simulink model "PV_fed_VCIMD_updated"  (R2019a)
settings: Solver=FixedStepAuto  StartTime=0.0  StopTime=20  RelTol=1e-3
undefined symbols (not defined in the file): L, Lm, Lr, Rr, sigbuilder_block
libraries: powerlib_meascontrol x17, powerlib x16, re_lib x1
settings Model: SimulationMode=accelerator  Creator=jetha  LastModifiedBy=HP
settings DataIOCC: ReturnWorkspaceOutputs=off
settings DebuggingCC: ArithmeticOperatorsInVariantConditions=warning

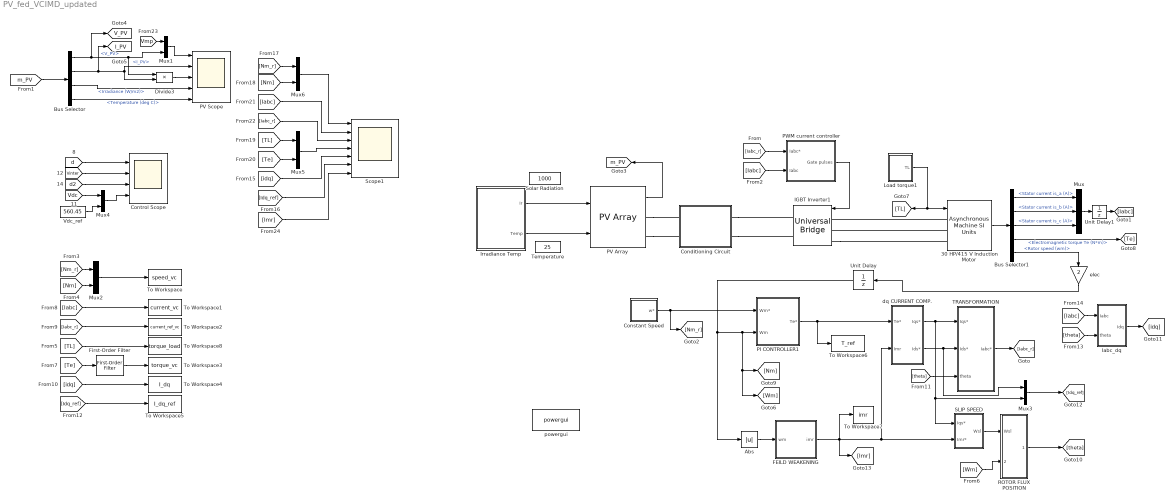
== system PV_fed_VCIMD_updated ==
  30 HP/415 V Induction Motor : powerlib/Machines/Asynchronous Machine SI Units  RotorType=Squirrel-cage  PresetModel=No  MechanicalLoad=Torque Tm  ShowDetailedParameters=on  ReferenceFrame=Rotor  Units=SI  MeasurementBus=off  NominalParameters=[30*746 415 50]  Stator=[0.251 0.001397]  Rotor=[Rr 0.001397]  Cage1=[ 0.022 0.226/377]  Cage2=[ 0.022 0.226/377]  Lm=0.0416  Mechanical=[0.305 0 2 ]  PolePairs=2  InitialConditions=[1 0 0 0 0 0 0 0]  SimulateSaturation=off  Saturation=[14.03593122, 27.81365428, 53.79336849, 72.68890987, 97.98006896, 148.6815601, 215.7428561, 302.9841135, 420.4778367 ; 230, 322, 414, 460, 506, 552, 598, 644, 690]  LoadFlowParameters=1492000  TsPowergui=0  TsBlock=-1  IterativeModel=Trapezoidal non iterative  IterativeDiscreteModel=Trapezoidal non iterative  Pmec=0
      settings: SourceProductName=Simscape Electrical
  Abs : Abs  SaturateOnIntegerOverflow=on
  Bus Selector : BusSelector  OutputSignals=V_PV,I_PV,Irradiance (W/m2),Temperature (deg C)
  Bus Selector1 : BusSelector  OutputSignals=Stator measurements.Stator current is_a (A),Stator measurements.Stator current is_b (A),Stator measurements.Stator current is_c (A),Mechanical.Electromagnetic torque Te (N*m),Mechanical.Rotor speed (wm)
  Conditioning Circuit : Subsystem
  Constant Speed : Subsystem
  Control Scope : Scope  NumInputPorts=4
  Divide3 : Product  Inputs=**
  FEILD WEAKENING : MATLAB Function  TreatAsAtomicUnit=on
  First-Order Filter : powerlib_meascontrol/Filters/First-Order Filter  FilterType=Lowpass  Tc=10e-3  Ts=0  Initialize=on  Vac_Init=[0, 0, 60]  Vdc_Init=0  PlotResponse=off  FreqRange="[0,  200,  1]"
      settings: SourceProductName=Simscape Electrical
  IGBT Inverter1 : powerlib/Power Electronics/Universal Bridge  Arms=3  SnubberResistance=1e5  SnubberCapacitance=inf  Device=MOSFET / Diodes  Ron=1e-3  Lon=0  ForwardVoltages="[  0  0  ]"  ForwardVoltage=0  GTOparameters=[ 10e-6 , 20e-6 ]  IGBTparameters=[ 1e-6 , 2e-6 ]  Measurements=None  Measurements_2=None  converterType=Rectifier
      settings: SourceProductName=Simscape Electrical
  Iabc_dq : Subsystem
  Irradiance Temp : Subsystem  Tag=STV Subsys  LoadFcn=sigbuilder_block('load');  StartFcn=sigbuilder_block('start');  StopFcn=sigbuilder_block('stop');  ClipboardFcn=sigbuilder_block('clipboard');  mask(Sigbuilder block){tuvar=[0:10]}
      mask help: Sigbuilder GUI
      mask init:
      | if ~strcmp(get_param(bdroot(gcbh),'SimulationStatus'),'stopped') tuvar = sigbuilder_block('maskInit'); end
      settings: CopyFcn=sigbuilder_block('copy');  DeleteFcn=sigbuilder_block('delete');  ModelCloseFcn=sigbuilder_block('modelClose');  PreSaveFcn=sigbuilder_block('preSave');  PauseFcn=sigbuilder_block('pause')  ContinueFcn=sigbuilder_block('continue')  NameChangeFcn=sigbuilder_block('namechange');  OpenFcn=sigbuilder_block('open',[87 109.8 1012.8 447.6 ]);  CloseFcn=sigbuilder_block('close');
      mask Display: plot(0, 0, 100, 100,[2, 2, 32, 32, 2], [68, 8, 8, 68, 68],[32, 2], [38, 38], [32, 19, 2],[53, 60, 44], [32, 17, 17, 2],[16, 16, 31, 31]);txt = getActiveGroup(gcbh);text(2, 100, txt,'verticalAlignment', 'top');
  Load torque1 : Subsystem
  Mux : Mux  Inputs=3
  Mux{1..6} (6 alike) : Mux  Inputs=2
  PI CONTROLLER1 : Subsystem  mask{Kp=120, Ki=2, Ts=100e-6, Lim=500}
      mask prompts: Ts "Sampling Time Ts (sec)"; Lim "Ref Torque limit(N-m)"
  PV Array : re_lib/Solar/PV Array  Npar=5  Nser=20  PlotType=array @ 25 deg.C & specified irradiances  S_vec=[ 1000 500 250 100 ]  Temp_C_vec="[ 25  50]"  ModuleName=Waaree Energies WSM-315  PlotWhenSelected=off  Pm=315  Ncell=72  Voc=43  Isc=9.77  Vm=35  Im=9  beta_Voc_pc=-0.338  alpha_Isc_pc=0.040901  beta_Voc=-0.14534  alpha_Isc=0.003996  IL=9.7966  I0=1.447e-10  nI=0.93356  Rsh=115.0566  Rs=0.31273  BAL=on  Tc=1e-6  Tfilter=5e-6
      settings: SourceProductName=Simscape Electrical
  PV Scope : Scope  NumInputPorts=5
  PWM current controller : Subsystem
  ROTOR FLUX POSITION : Subsystem
  SLIP SPEED : Subsystem
  Scope1 : Scope  NumInputPorts=7
  Solar Radiation : Constant  Value=1000
  TRANSFORMATION : Subsystem
  Temperature : Constant  Value=25
  To Workspace : ToWorkspace  VariableName=speed_vc  SaveFormat=Structure With Time  SampleTime=100e-6
  To Workspace1 : ToWorkspace  VariableName=current_vc  SaveFormat=Structure With Time  SampleTime=100e-6
  To Workspace2 : ToWorkspace  VariableName=current_ref_vc  SaveFormat=Structure With Time  SampleTime=100e-6
  To Workspace3 : ToWorkspace  VariableName=torque_vc  SaveFormat=Structure With Time  SampleTime=100e-6
  To Workspace4 : ToWorkspace  VariableName=I_dq  SaveFormat=Structure With Time  SampleTime=100e-6
  To Workspace5 : ToWorkspace  VariableName=I_dq_ref  SaveFormat=Structure With Time  SampleTime=100e-6
  To Workspace6 : ToWorkspace  VariableName=T_ref  SaveFormat=Structure With Time  SampleTime=100e-6
  To Workspace7 : ToWorkspace  VariableName=imr  SaveFormat=Structure With Time  SampleTime=100e-6
  To Workspace8 : ToWorkspace  VariableName=torque_load  SaveFormat=Structure With Time  SampleTime=100e-6
  Unit Delay : UnitDelay  SampleTime=100e-6  HasFrameUpgradeWarning=on
  Unit Delay1 : UnitDelay  SampleTime=10e-6  HasFrameUpgradeWarning=on
  Vdc_ref : Constant  Value=560.45
  dq CURRENT COMP. : Subsystem
  elec : Gain  Gain=2
  powergui : powerlib/powergui  Priority=1  SimulationMode=Discrete  SampleTime=1e-5  frequency=60  Iterations=50  frequencyindice=0  Pbase=100e6  ErrMax=1e-4  UnitsV=kV  UnitsW=MW  buscounter=0  FunctionMessages=off  echomessages=off  EnableUseOfTLC=off  CurrentSourceSwitches=off  DisableSnubberDevices=off  DisableRonSwitches=off  DisableVfSwitches=off  DisplayEquations=off  AutomaticDiscreteSolvers=off  SolverType=Tustin/Backward Euler (TBE)  Interpol=off  ExternalGateDelay=off  methode=off  Ts=100  x0status=blocks  SPID=off  SwTol=0  HookPort=off  NonlinearTolerance=0  nMaxIteration=15  ContinueOnMaxIteration=off  RestoreLinks=warning  ResistiveCurrentMeasurement=off  Frange=[0:2:500]  Ylog=off  Xlog=on  ShowGrid=off  save=off  variable=ZData  structure=0  ZoomFFT=off  StartTime=0.0  cycles=1  DisplayStyle=1  fundamental=60  FreqAxis=off  MaxFrequency=1000  frequencyindicesteady=1  RmsSteady=1  display=off
      settings: SourceProductName=Simscape Electrical
  tag scope: I_PV=global, V_PV=global, m_PV=global
  wires:
  PV Array/1 -> [m_PV]
  Load torque1/1(TL) -> 30 HP/415 V Induction Motor/1, [TL]
  [theta] -> Iabc_dq/2(theta)
  [Iabc] -> Iabc_dq/1(Iabc)
  SLIP SPEED/1(Wsl) -> ROTOR FLUX POSITION/1("Wsl\t")
  elec/1 -> Unit Delay/1
  [theta] -> TRANSFORMATION/3(theta)
  [Iabc_r] -> PWM current controller/1(Iabc*)
  [Wm] -> ROTOR FLUX POSITION/2(Wm)
  Bus Selector1/4 -> [Te]  "<Electromagnetic torque Te (N*m)>"
  ROTOR FLUX POSITION/1(theta) -> [theta]
  dq CURRENT COMP./1(Iqs*) -> TRANSFORMATION/1(Iqs*), SLIP SPEED/1(Iqs*), Mux3/2
  Mux3/1 -> [Idq_ref]
  Abs/1 -> FEILD WEAKENING/1(wm)
  Unit Delay1/1 -> [Iabc]
  Iabc_dq/1(Idq) -> [idq]
  PWM current controller/1(Gate pulses) -> IGBT Inverter1/1
  Bus Selector1/5 -> elec/1  "<Rotor speed (wm)>"
  30 HP/415 V Induction Motor/1 -> Bus Selector1/1
  Mux/1 -> Unit Delay1/1
  dq CURRENT COMP./2(Ids*) -> Mux3/1, TRANSFORMATION/2(Ids*)
  Bus Selector1/1 -> Mux/1  "<Stator current is_a (A)>"
  FEILD WEAKENING/1(imr) -> [Imr], dq CURRENT COMP./2(Imr), SLIP SPEED/2(Imr*), To Workspace7/1
  Unit Delay/1 -> Abs/1, PI CONTROLLER1/2(Wm), [Nm], [Wm]
  Bus Selector1/2 -> Mux/2  "<Stator current is_b (A)>"
  TRANSFORMATION/1(Iabc*) -> [Iabc_r]
  PI CONTROLLER1/1(Te*) -> To Workspace6/1, dq CURRENT COMP./1(Te*)
  Bus Selector1/3 -> Mux/3  "<Stator current is_c (A)>"
  [Iabc] -> PWM current controller/2(Iabc)
  Constant Speed/1(w*) -> PI CONTROLLER1/1(Wm*), [Nm_r]
  Irradiance Temp/1(Ir) -> PV Array/1
  Irradiance Temp/2(Temp) -> PV Array/2
  [d] -> Control Scope/1
  [Iabc] -> Scope1/2
  [Te] -> First-Order Filter/1
  Mux2/1 -> To Workspace/1
  [Iabc] -> To Workspace1/1
  [Nm] -> Mux2/2
  Vdc_ref/1 -> Mux4/2
  Mux4/1 -> Control Scope/4
  Mux5/1 -> Scope1/4
  [Idq_ref] -> To Workspace5/1
  Bus Selector/3 -> PV Scope/4  "<Irradiance (W/m2)>"
  [Vdc] -> Mux4/1
  Mux1/1 -> PV Scope/1
  [idq] -> Scope1/5
  Bus Selector/2 -> [I_PV], PV Scope/2, Divide3/2  "<I_PV>"
  [d2] -> Control Scope/3
  Divide3/1 -> PV Scope/3
  [TL] -> To Workspace8/1
  [Te] -> Mux5/2
  Bus Selector/4 -> PV Scope/5  "<Temperature (deg C)>"
  [TL] -> Mux5/1
  [Nm] -> Mux6/2
  [m_PV] -> Bus Selector/1
  Mux6/1 -> Scope1/1
  [Iabc_r] -> Scope1/3
  Bus Selector/1 -> [V_PV], Mux1/2, Divide3/1  "<V_PV>"
  [idq] -> To Workspace4/1
  [Iabc_r] -> To Workspace2/1
  [Idq_ref] -> Scope1/6
  [Nm_r] -> Mux2/1
  First-Order Filter/1 -> To Workspace3/1
  [Nm_r] -> Mux6/1
  [Vinter] -> Control Scope/2
  [Vmp] -> Mux1/1
  [Imr] -> Scope1/7
  connections:
  PV Array/RConn1 -- Conditioning Circuit/LConn1
  PV Array/RConn2 -- Conditioning Circuit/LConn2
  30 HP/415 V Induction Motor/LConn1 -- IGBT Inverter1/LConn1
  IGBT Inverter1/LConn3 -- 30 HP/415 V Induction Motor/LConn3
  30 HP/415 V Induction Motor/LConn2 -- IGBT Inverter1/LConn2
  Conditioning Circuit/RConn1 -- IGBT Inverter1/RConn1
  Conditioning Circuit/RConn2 -- IGBT Inverter1/RConn2

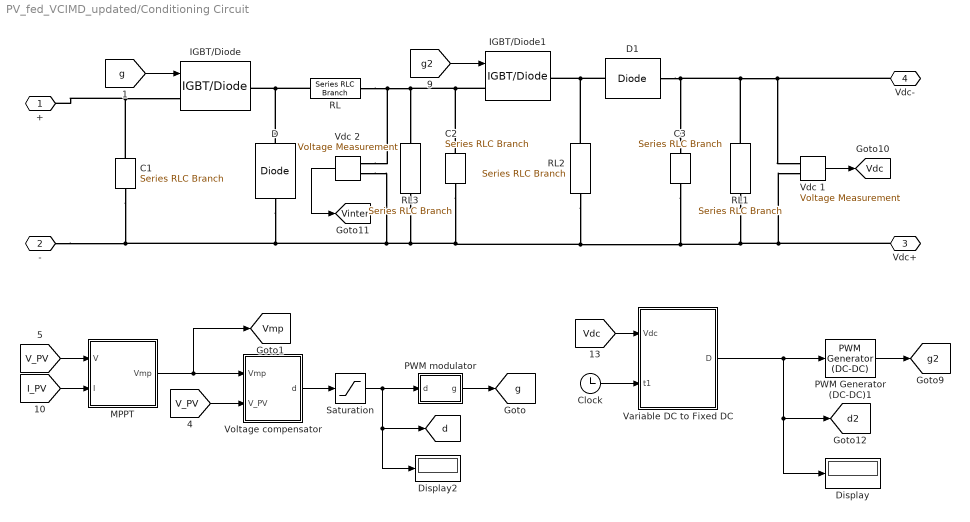
== system PV_fed_VCIMD_updated/Conditioning Circuit ==
  C1 : powerlib/Elements/Series RLC Branch  LConnTagsString=__new0  RConnTagsString=__new0  BranchType=C  Resistance=1  Inductance=L  SetiL0=off  InitialCurrent=0  Capacitance=1e-3  Setx0=off  InitialVoltage=Vmp  Measurements=None
      settings: SourceProductName=Simscape Electrical
  C2 : powerlib/Elements/Series RLC Branch  LConnTagsString=__new0  RConnTagsString=__new0  BranchType=C  Resistance=1  Inductance=L  SetiL0=off  InitialCurrent=0  Capacitance=5e-3  Setx0=off  InitialVoltage=Vmp  Measurements=None
      settings: SourceProductName=Simscape Electrical
  C3 : powerlib/Elements/Series RLC Branch  LConnTagsString=__new0  RConnTagsString=__new0  BranchType=C  Resistance=1  Inductance=L  SetiL0=off  InitialCurrent=0  Capacitance=5e-2  Setx0=off  InitialVoltage=Vmp  Measurements=None
      settings: SourceProductName=Simscape Electrical
  Clock : Clock
  D : powerlib/Power Electronics/Diode  Ron=1e-4  Lon=0  Vf=0  IC=0  UseSnubber=off  Rs=inf  Cs=inf  Measurements=off
      settings: SourceProductName=Simscape Electrical
  D1 : powerlib/Power Electronics/Diode  Ron=1e-4  Lon=0  Vf=0  IC=0  UseSnubber=off  Rs=inf  Cs=inf  Measurements=off
      settings: SourceProductName=Simscape Electrical
  Display : Display
  Display2 : Display
  IGBT/Diode : powerlib/Power Electronics/IGBT//Diode  Ron=1e-3  Rs=1e5  Cs=inf  Measurements=off
      settings: SourceProductName=Simscape Electrical
  IGBT/Diode1 : powerlib/Power Electronics/IGBT//Diode  Ron=1e-3  Rs=1e5  Cs=inf  Measurements=off
      settings: SourceProductName=Simscape Electrical
  MPPT : MATLAB Function  TreatAsAtomicUnit=on
  PWM modulator : Subsystem
  PWM Generator (DC-DC)1 : powerlib_meascontrol/Pulse & Signal Generators/PWM Generator (DC-DC)  Fsw=10000  Ts=0
      settings: SourceProductName=Simscape Electrical
  RL : powerlib/Elements/Series RLC Branch  LConnTagsString=__new0  RConnTagsString=__new0  BranchType=RL  Resistance=5e-3  Inductance=0.01  SetiL0=off  InitialCurrent=0  Capacitance=1e-6  Setx0=off  InitialVoltage=0  Measurements=None
      settings: SourceProductName=Simscape Electrical
  RL1 : powerlib/Elements/Series RLC Branch  LConnTagsString=__new0  RConnTagsString=__new0  BranchType=R  Resistance=150  Inductance=10e-3  SetiL0=off  InitialCurrent=0  Capacitance=1e-6  Setx0=off  InitialVoltage=0  Measurements=None
      settings: SourceProductName=Simscape Electrical
  RL2 : powerlib/Elements/Series RLC Branch  LConnTagsString=__new0  RConnTagsString=__new0  BranchType=RL  Resistance=5e-3  Inductance=1e-2  SetiL0=off  InitialCurrent=0  Capacitance=1e-6  Setx0=off  InitialVoltage=0  Measurements=None
      settings: SourceProductName=Simscape Electrical
  RL3 : powerlib/Elements/Series RLC Branch  LConnTagsString=__new0  RConnTagsString=__new0  BranchType=R  Resistance=5  Inductance=10e-3  SetiL0=off  InitialCurrent=0  Capacitance=1e-6  Setx0=off  InitialVoltage=0  Measurements=None
      settings: SourceProductName=Simscape Electrical
  Saturation : Saturate  UpperLimit=0.9  LowerLimit=0.1  LinearizeAsGain=off
  Variable DC to Fixed DC : MATLAB Function  TreatAsAtomicUnit=on
  Vdc 1 : powerlib/Measurements/Voltage Measurement  Tag=PoWeRsYsTeMmEaSuReMeNt  PhasorSimulation=off  OutputType=Magnitude  PSBequivalent=0
      settings: SourceProductName=Simscape Electrical
  Vdc 2 : powerlib/Measurements/Voltage Measurement  Tag=PoWeRsYsTeMmEaSuReMeNt  PhasorSimulation=off  OutputType=Magnitude  PSBequivalent=0
      settings: SourceProductName=Simscape Electrical
  Voltage compensator : Subsystem
  + : PMIOPort  Side=Left
  - : PMIOPort  Port=2  Side=Left
  Vdc+ : PMIOPort  Port=3  Side=Right
  Vdc- : PMIOPort  Port=4  Side=Right
  tag scope: Vdc=global, Vinter=global, Vmp=global, d2=global, d=global, g2=global, g=global
  wires:
  PWM Generator (DC-DC)1/1 -> [g2]
  [Vdc] -> Variable DC to Fixed DC/1(Vdc)
  Variable DC to Fixed DC/1(D) -> Display/1, [d2], PWM Generator (DC-DC)1/1
  Clock/1 -> Variable DC to Fixed DC/2(t1)
  [V_PV] -> Voltage compensator/2(V_PV)
  [I_PV] -> MPPT/2(I)
  [V_PV] -> MPPT/1(V)
  PWM modulator/1(g) -> [g]
  MPPT/1(Vmp) -> [Vmp], Voltage compensator/1(Vmp)
  Voltage compensator/1(d) -> Saturation/1
  Saturation/1 -> Display2/1, [d], PWM modulator/1(d)
  Vdc 2/1 -> [Vinter]
  Vdc 1/1 -> [Vdc]
  [g2] -> IGBT/Diode1/1
  [g] -> IGBT/Diode/1
  connections:
  C3/RConn1 -- Vdc+/RConn1 -- Vdc 1/LConn1 -- RL1/RConn1 -- RL2/RConn1 -- RL3/RConn1 -- D/LConn1 -- -/RConn1 -- C1/RConn1 -- Vdc 2/LConn2 -- C2/RConn1
  C3/LConn1 -- Vdc 1/LConn2 -- Vdc-/RConn1 -- RL1/LConn1 -- D1/LConn1
  +/RConn1 -- C1/LConn1 -- IGBT/Diode/LConn1
  Vdc 2/LConn1 -- RL/LConn1 -- RL3/LConn1 -- C2/LConn1 -- IGBT/Diode1/LConn1
  IGBT/Diode/RConn1 -- D/RConn1 -- RL/RConn1
  IGBT/Diode1/RConn1 -- RL2/LConn1 -- D1/RConn1

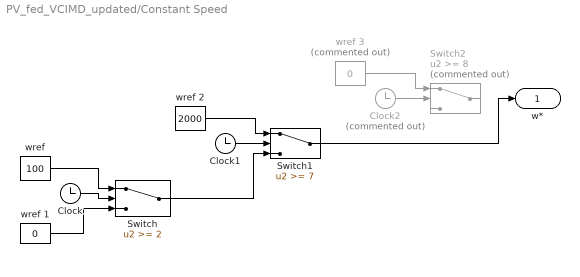
== system PV_fed_VCIMD_updated/Constant Speed ==
  Clock : Clock
      settings: Decimation=2
  Clock1 : Clock
      settings: Decimation=2
  Clock2 : Clock  Commented=on
      settings: Decimation=2
  Switch : Switch  Threshold=2  SaturateOnIntegerOverflow=on  InputSameDT=on
  Switch1 : Switch  Threshold=7  SaturateOnIntegerOverflow=on  InputSameDT=on
  Switch2 : Switch  Commented=on  Threshold=8  SaturateOnIntegerOverflow=on  InputSameDT=on
  "wref " : Constant  Value=100
  wref 1 : Constant  Value=0
  wref 2 : Constant  Value=2000  VectorParams1D=off
  wref 3 : Constant  Commented=on  Value=0  VectorParams1D=off
  w* : Outport
  wires:
  wref 1/1 -> Switch/3
  Clock/1 -> Switch/2
  "wref "/1 -> Switch/1
  wref 2/1 -> Switch1/1
  Clock1/1 -> Switch1/2
  Switch/1 -> Switch1/3
  wref 3/1 -> Switch2/1
  Clock2/1 -> Switch2/2
  Switch1/1 -> w*/1

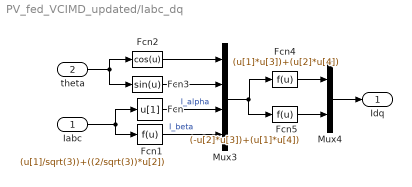
== system PV_fed_VCIMD_updated/Iabc_dq ==
  Iabc : Inport
  theta : Inport  Port=2
  Fcn : Fcn  Expr=u[1]
  Fcn1 : Fcn  Expr=(u[1]/sqrt(3))+((2/sqrt(3))*u[2])
  Fcn2 : Fcn  Expr=cos(u)
  Fcn3 : Fcn  Expr=sin(u)
  Fcn4 : Fcn  Expr=(u[1]*u[3])+(u[2]*u[4])
  Fcn5 : Fcn  Expr=(-u[2]*u[3])+(u[1]*u[4])
  Mux3 : Mux
  Mux4 : Mux  Inputs=2
  Idq : Outport
  wires:
  Iabc/1 -> Fcn1/1, Fcn/1
  theta/1 -> Fcn2/1, Fcn3/1
  Fcn2/1 -> Mux3/1
  Fcn3/1 -> Mux3/2
  Fcn/1 -> Mux3/3  "I_alpha"
  Mux3/1 -> Fcn5/1, Fcn4/1
  Fcn4/1 -> Mux4/1
  Fcn5/1 -> Mux4/2
  Mux4/1 -> Idq/1
  Fcn1/1 -> Mux3/4  "I_beta"

== system PV_fed_VCIMD_updated/Irradiance Temp ==
  Demux : Demux  Tag=STV Demux  Outputs=2
  FromWs : FromWorkspace  Tag=STV FromWs  VariableName=tuvar  SampleTime=0
      SigBuilderData=|
      | common.afterFinalStr = 'Extrapolate'
      | common.sampleTime = '0'
      | dataSet(1).timeRange = [0 6]
      | dataSet(1).name = 'Constant Irradiance'
      | dataSet(2).timeRange = [0 20]
      | dataSet(2).name = 'Ramp-up/down Irradiance'
      | dataSet(3).timeRange = [0 6]
      | dataSet(3).name = 'Step Irradiance'
      | sbobj.Groups(1).Name = 'Constant Irradiance'
      | sbobj.Groups(1).Signals(1).Name = 'Ir'
      | sbobj.Groups(1).Signals(1).XData = [0 6]
      | sbobj.Groups(1).Signals(1).YData = [1000 1000]
      | sbobj.Groups(1).Signals(2).Name = 'Temp'
      | sbobj.Groups(1).Signals(2).XData = [0 2.4 2.4 3.6 3.6 6]
      | sbobj.Groups(1).Signals(2).YData = [0 0 1 1 0 0]
      | sbobj.Groups(1).TimeRange = [0 6]
      | sbobj.Groups(2).Name = 'Ramp-up/down Irradiance'
      | sbobj.Groups(2).Signals(1).Name = 'Ir'
      | sbobj.Groups(2).Signals(1).XData = [0 3 3.5 4 4.5 20]
      | sbobj.Groups(2).Signals(1).YData = [1000 1000 400 400 1000 1000]
      | sbobj.Groups(2).Signals(2).Name = 'Temp'
      | sbobj.Groups(2).Signals(2).XData = [0 5 5.5 6 6.5 20]
      | sbobj.Groups(2).Signals(2).YData = [25 25 50 50 25 25]
      | sbobj.Groups(2).TimeRange = [0 20]
      | sbobj.Groups(3).Name = 'Step Irradiance'
      | sbobj.Groups(3).Signals(1).Name = 'Ir'
      | sbobj.Groups(3).Signals(1).XData = [0 0.252 0.252 6]
      | sbobj.Groups(3).Signals(1).YData = [600 600 1000 1000]
      | sbobj.Groups(3).Signals(2).Name = 'Temp'
      | sbobj.Groups(3).Signals(2).XData = [0 2.4 2.4 3.6 3.6 6]
      | sbobj.Groups(3).Signals(2).YData = [0 0 1 1 0 0]
      | sbobj.Groups(3).TimeRange = [0 6]
  Ir : Outport  Tag=STV Outport
  Temp : Outport  Tag=STV Outport  Port=2
  wires:
  Demux/1 -> Ir/1
  FromWs/1 -> Demux/1
  Demux/2 -> Temp/1

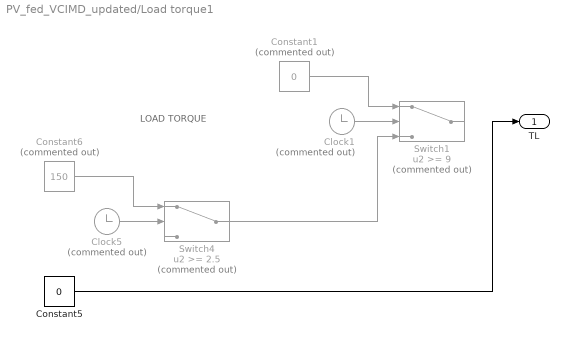
== system PV_fed_VCIMD_updated/Load torque1 ==
  note: LOAD TORQUE
  Clock1 : Clock  Commented=on
  Clock5 : Clock  Commented=on
  Constant1 : Constant  Commented=on  Value=0
  Constant5 : Constant  Value=0
  Constant6 : Constant  Commented=on  Value=150
  Switch1 : Switch  Commented=on  Threshold=9
  Switch4 : Switch  Commented=on  Threshold=2.5
  TL : Outport
  wires:
  Constant5/1 -> TL/1
  Constant6/1 -> Switch4/1
  Clock5/1 -> Switch4/2
  Constant1/1 -> Switch1/1
  Clock1/1 -> Switch1/2
  Switch4/1 -> Switch1/3

== system PV_fed_VCIMD_updated/PI CONTROLLER1 ==
  note: Wm*
  note: Wm
  Wm* : Inport
  Wm : Inport  Port=2
  Subsystem : Subsystem
  Sum : Sum  Inputs=|+-
  Te* : Outport
  wires:
  Wm*/1 -> Sum/1
  Subsystem/1(Te*) -> Te*/1
  Sum/1 -> Subsystem/1(We)
  Wm/1 -> Sum/2

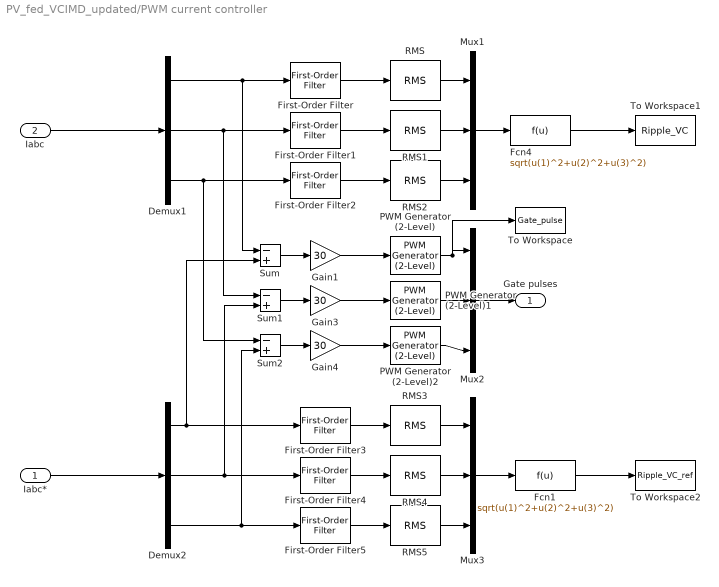
== system PV_fed_VCIMD_updated/PWM current controller ==
  Iabc* : Inport
  Iabc : Inport  Port=2
  Demux1 : Demux  Outputs=3
  Demux2 : Demux  Outputs=3
  Fcn1 : Fcn  Expr=sqrt(u(1)^2+u(2)^2+u(3)^2)
  Fcn4 : Fcn  Expr=sqrt(u(1)^2+u(2)^2+u(3)^2)
  First-Order Filter : powerlib_meascontrol/Filters/First-Order Filter  FilterType=Highpass  Tc=0.5e-3  Ts=0  Initialize=on  Vac_Init=[0, 0, 60]  Vdc_Init=0  PlotResponse=off  FreqRange="[0,  200,  1]"
      settings: SourceProductName=Simscape Electrical
  First-Order Filter1 : powerlib_meascontrol/Filters/First-Order Filter  FilterType=Highpass  Tc=0.5e-3  Ts=0  Initialize=on  Vac_Init=[0, 0, 60]  Vdc_Init=0  PlotResponse=off  FreqRange="[0,  200,  1]"
      settings: SourceProductName=Simscape Electrical
  First-Order Filter2 : powerlib_meascontrol/Filters/First-Order Filter  FilterType=Highpass  Tc=0.5e-3  Ts=0  Initialize=on  Vac_Init=[0, 0, 60]  Vdc_Init=0  PlotResponse=off  FreqRange="[0,  200,  1]"
      settings: SourceProductName=Simscape Electrical
  First-Order Filter3 : powerlib_meascontrol/Filters/First-Order Filter  FilterType=Highpass  Tc=0.5e-3  Ts=0  Initialize=on  Vac_Init=[0, 0, 50]  Vdc_Init=0  PlotResponse=off  FreqRange="[0,  200,  1]"
      settings: SourceProductName=Simscape Electrical
  First-Order Filter4 : powerlib_meascontrol/Filters/First-Order Filter  FilterType=Highpass  Tc=0.5e-3  Ts=0  Initialize=on  Vac_Init=[0, 0, 50]  Vdc_Init=0  PlotResponse=off  FreqRange="[0,  200,  1]"
      settings: SourceProductName=Simscape Electrical
  First-Order Filter5 : powerlib_meascontrol/Filters/First-Order Filter  FilterType=Highpass  Tc=0.5e-3  Ts=0  Initialize=on  Vac_Init=[0, 0, 50]  Vdc_Init=0  PlotResponse=off  FreqRange="[0,  200,  1]"
      settings: SourceProductName=Simscape Electrical
  Gain1 : Gain  Gain=30  SaturateOnIntegerOverflow=on  OutDataTypeStr=Inherit: Same as input  ParamDataTypeStr=Inherit: Same as input
  Gain3 : Gain  Gain=30  SaturateOnIntegerOverflow=on  OutDataTypeStr=Inherit: Same as input  ParamDataTypeStr=Inherit: Same as input
  Gain4 : Gain  Gain=30  SaturateOnIntegerOverflow=on  OutDataTypeStr=Inherit: Same as input  ParamDataTypeStr=Inherit: Same as input
  Mux1 : Mux  Inputs=3
  Mux2 : Mux  Inputs=3
  Mux3 : Mux  Inputs=3
  PWM Generator (2-Level) : powerlib_meascontrol/Pulse & Signal Generators/PWM Generator (2-Level)  ModulatorType=Single-phase half-bridge (2 pulses)  ModulatorMode=Unsynchronized  Fc=10000  Pc=90  nF=27  MinMax="[ -1  1 ]"  SamplingTechnique=Natural  ModulatingSignals=off  m=0.8  Freq=60  Phase=0  Ts=10e-6  ShowCarrierOutport=off
  PWM Generator (2-Level)1 : powerlib_meascontrol/Pulse & Signal Generators/PWM Generator (2-Level)  ModulatorType=Single-phase half-bridge (2 pulses)  ModulatorMode=Unsynchronized  Fc=10000  Pc=90  nF=27  MinMax="[ -1  1 ]"  SamplingTechnique=Natural  ModulatingSignals=off  m=0.8  Freq=60  Phase=0  Ts=5e-6  ShowCarrierOutport=off
  PWM Generator (2-Level)2 : powerlib_meascontrol/Pulse & Signal Generators/PWM Generator (2-Level)  ModulatorType=Single-phase half-bridge (2 pulses)  ModulatorMode=Unsynchronized  Fc=10000  Pc=90  nF=27  MinMax="[ -1  1 ]"  SamplingTechnique=Natural  ModulatingSignals=off  m=0.8  Freq=60  Phase=0  Ts=5e-6  ShowCarrierOutport=off
  RMS : powerlib_meascontrol/Measurements/RMS  TrueRMS=on  Freq=60  RMSInit=120  Ts=0
      settings: SourceProductName=Simscape Electrical
  RMS1 : powerlib_meascontrol/Measurements/RMS  TrueRMS=on  Freq=60  RMSInit=120  Ts=0
      settings: SourceProductName=Simscape Electrical
  RMS2 : powerlib_meascontrol/Measurements/RMS  TrueRMS=on  Freq=60  RMSInit=120  Ts=0
      settings: SourceProductName=Simscape Electrical
  RMS3 : powerlib_meascontrol/Measurements/RMS  TrueRMS=off  Freq=50  RMSInit=0  Ts=0
      settings: SourceProductName=Simscape Electrical
  RMS4 : powerlib_meascontrol/Measurements/RMS  TrueRMS=off  Freq=50  RMSInit=0  Ts=0
      settings: SourceProductName=Simscape Electrical
  RMS5 : powerlib_meascontrol/Measurements/RMS  TrueRMS=off  Freq=50  RMSInit=0  Ts=0
      settings: SourceProductName=Simscape Electrical
  Sum : Sum  Inputs=-+  SaturateOnIntegerOverflow=on  InputSameDT=on  OutDataTypeStr=Inherit: Same as first input
  Sum1 : Sum  Inputs=-+  SaturateOnIntegerOverflow=on  InputSameDT=on  OutDataTypeStr=Inherit: Same as first input
  Sum2 : Sum  Inputs=-+  SaturateOnIntegerOverflow=on  InputSameDT=on  OutDataTypeStr=Inherit: Same as first input
  To Workspace : ToWorkspace  VariableName=Gate_pulse  SaveFormat=Structure With Time  SampleTime=100e-6
  To Workspace1 : ToWorkspace  VariableName=Ripple_VC  SaveFormat=Structure With Time  SampleTime=100e-6
  To Workspace2 : ToWorkspace  VariableName=Ripple_VC_ref  SaveFormat=Structure With Time  SampleTime=100e-6
  Gate pulses : Outport
  wires:
  PWM Generator (2-Level)/1 -> To Workspace/1, Mux2/1
  PWM Generator (2-Level)1/1 -> Mux2/2
  PWM Generator (2-Level)2/1 -> Mux2/3
  Gain3/1 -> PWM Generator (2-Level)1/1
  Gain4/1 -> PWM Generator (2-Level)2/1
  Mux2/1 -> Gate pulses/1
  Gain1/1 -> PWM Generator (2-Level)/1
  Demux1/1 -> Sum/1, First-Order Filter/1
  Iabc/1 -> Demux1/1
  Demux1/3 -> First-Order Filter2/1, Sum2/1
  Iabc*/1 -> Demux2/1
  Sum/1 -> Gain1/1
  Sum1/1 -> Gain3/1
  Sum2/1 -> Gain4/1
  Demux1/2 -> First-Order Filter1/1, Sum1/1
  First-Order Filter/1 -> RMS/1
  First-Order Filter1/1 -> RMS1/1
  First-Order Filter2/1 -> RMS2/1
  RMS2/1 -> Mux1/3
  RMS1/1 -> Mux1/2
  RMS/1 -> Mux1/1
  Mux1/1 -> Fcn4/1
  Fcn4/1 -> To Workspace1/1
  Demux2/1 -> First-Order Filter3/1, Sum/2
  Demux2/2 -> First-Order Filter4/1, Sum1/2
  Demux2/3 -> Sum2/2, First-Order Filter5/1
  RMS5/1 -> Mux3/3
  RMS4/1 -> Mux3/2
  RMS3/1 -> Mux3/1
  Mux3/1 -> Fcn1/1
  Fcn1/1 -> To Workspace2/1
  First-Order Filter3/1 -> RMS3/1
  First-Order Filter4/1 -> RMS4/1
  First-Order Filter5/1 -> RMS5/1

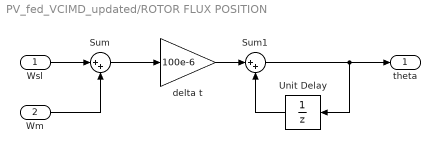
== system PV_fed_VCIMD_updated/ROTOR FLUX POSITION ==
  "Wsl\t" : Inport
  Wm : Inport  Port=2
  Sum : Sum  Inputs=|++
  Sum1 : Sum  Inputs=|++
  Unit Delay : UnitDelay  SampleTime=100e-6  HasFrameUpgradeWarning=on
  delta t : Gain  Gain=100e-6
  theta : Outport
  wires:
  delta t/1 -> Sum1/1
  Sum1/1 -> theta/1, Unit Delay/1
  Sum/1 -> delta t/1
  Unit Delay/1 -> Sum1/2
  Wm/1 -> Sum/2
  "Wsl\t"/1 -> Sum/1

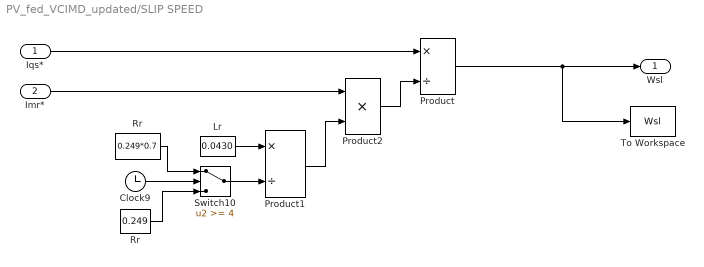
== system PV_fed_VCIMD_updated/SLIP SPEED ==
  Iqs* : Inport
  Imr* : Inport  Port=2
  Clock9 : Clock
      settings: Decimation=2
  Lr : Constant  Value=0.0430
  Product : Product  Inputs=*/
  Product1 : Product  Inputs=*/
  Product2 : Product  Inputs=**
  Rr : Constant  Value=0.249*0.7
  "Rr " : Constant  Value=0.249
  Switch10 : Switch  Threshold=4  SaturateOnIntegerOverflow=on  InputSameDT=on
  To Workspace : ToWorkspace  VariableName=Wsl  SaveFormat=Structure With Time  SampleTime=100e-6
  Wsl : Outport
  wires:
  Iqs*/1 -> Product/1
  Product2/1 -> Product/2
  Imr*/1 -> Product2/1
  Clock9/1 -> Switch10/2
  "Rr "/1 -> Switch10/3
  Rr/1 -> Switch10/1
  Switch10/1 -> Product1/2
  Lr/1 -> Product1/1
  Product1/1 -> Product2/2
  Product/1 -> To Workspace/1, Wsl/1

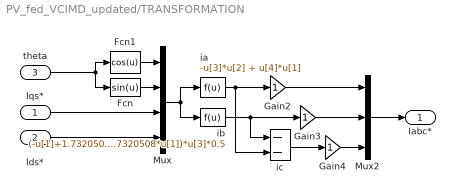
== system PV_fed_VCIMD_updated/TRANSFORMATION ==
  Iqs* : Inport
  Ids* : Inport  Port=2
  theta : Inport  Port=3
  Fcn : Fcn  Expr=sin(u)
  Fcn1 : Fcn  Expr=cos(u)
  Gain2 : Gain  SaturateOnIntegerOverflow=on  OutDataTypeStr=Inherit: Same as input  ParamDataTypeStr=Inherit: Same as input
  Gain3 : Gain  SaturateOnIntegerOverflow=on  OutDataTypeStr=Inherit: Same as input  ParamDataTypeStr=Inherit: Same as input
  Gain4 : Gain  SaturateOnIntegerOverflow=on  OutDataTypeStr=Inherit: Same as input  ParamDataTypeStr=Inherit: Same as input
  Mux : Mux
  Mux2 : Mux  Inputs=3
  ia : Fcn  Expr=-u[3]*u[2] + u[4]*u[1]
  ib : Fcn  Expr=(-u[1]+1.7320508*u[2])*u[4]*0.5+(u[2]+1.7320508*u[1])*u[3]*0.5
  ic : Sum  Inputs=--  SaturateOnIntegerOverflow=on  InputSameDT=on  OutDataTypeStr=Inherit: Same as first input
  Iabc* : Outport
  wires:
  Fcn/1 -> Mux/2
  theta/1 -> Fcn/1, Fcn1/1
  Mux2/1 -> Iabc*/1
  Gain3/1 -> Mux2/2
  Fcn1/1 -> Mux/1
  ic/1 -> Gain4/1
  ib/1 -> Gain3/1, ic/1
  Mux/1 -> ia/1, ib/1
  ia/1 -> Gain2/1, ic/2
  Iqs*/1 -> Mux/3
  Ids*/1 -> Mux/4
  Gain2/1 -> Mux2/1
  Gain4/1 -> Mux2/3

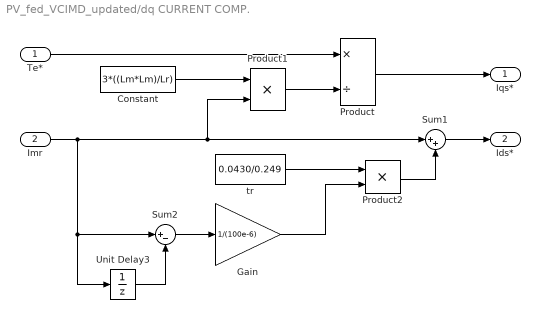
== system PV_fed_VCIMD_updated/dq CURRENT COMP. ==
  Te* : Inport
  Imr : Inport  Port=2
  Constant : Constant  Value=3*((Lm*Lm)/Lr)
  Gain : Gain  Gain=1/(100e-6)
  Product : Product  Inputs=*/
  Product1 : Product
  Product2 : Product  SaturateOnIntegerOverflow=on  InputSameDT=on  OutDataTypeStr=Inherit: Same as first input
  Sum1 : Sum  Inputs=|++
  Sum2 : Sum  Inputs=|+-
  Unit Delay3 : UnitDelay  SampleTime=100e-6  HasFrameUpgradeWarning=on
  tr : Constant  Value=0.0430/0.249
  Iqs* : Outport
  Ids* : Outport  Port=2
  wires:
  Product1/1 -> Product/2
  Constant/1 -> Product1/1
  Te*/1 -> Product/1
  Product/1 -> Iqs*/1
  Imr/1 -> Product1/2, Sum1/1, Unit Delay3/1, Sum2/1
  tr/1 -> Product2/1
  Product2/1 -> Sum1/2
  Sum1/1 -> Ids*/1
  Unit Delay3/1 -> Sum2/2
  Sum2/1 -> Gain/1
  Gain/1 -> Product2/2

== system PV_fed_VCIMD_updated/Conditioning Circuit/PWM modulator ==
  d : Inport
  Comparator : Subsystem
      settings: RTWSystemCode=Inline
  Sawtooth : Subsystem
  g : Outport
  wires:
  Sawtooth/1(Out1) -> Comparator/2(In2)
  d/1 -> Comparator/1(In1)
  Comparator/1(Out1) -> g/1

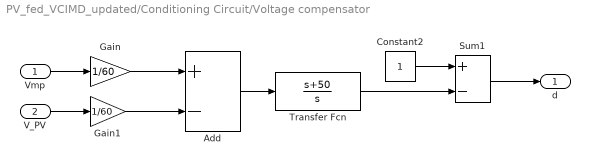
== system PV_fed_VCIMD_updated/Conditioning Circuit/Voltage compensator ==
  Vmp : Inport
  V_PV : Inport  Port=2
  Add : Sum  Inputs=+-
  Constant2 : Constant
  Gain : Gain  Gain=1/60
  Gain1 : Gain  Gain=1/60
  Sum1 : Sum  Inputs=+-
  Transfer Fcn : TransferFcn  Numerator=[1 50]  Denominator=[1 0]
  d : Outport
  wires:
  Vmp/1 -> Gain/1
  V_PV/1 -> Gain1/1
  Add/1 -> Transfer Fcn/1
  Constant2/1 -> Sum1/1
  Transfer Fcn/1 -> Sum1/2
  Sum1/1 -> d/1
  Gain/1 -> Add/1
  Gain1/1 -> Add/2

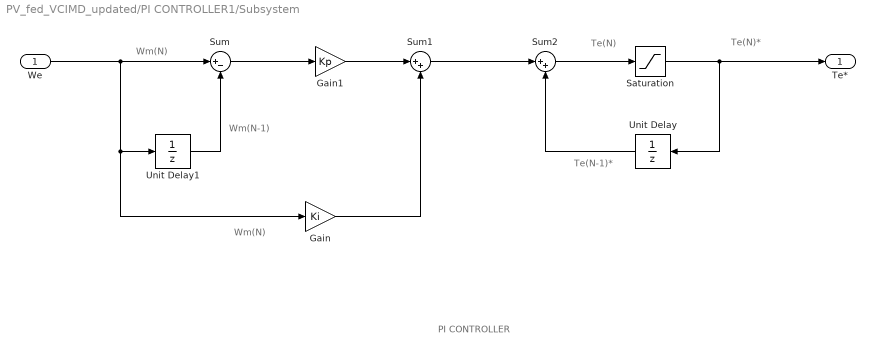
== system PV_fed_VCIMD_updated/PI CONTROLLER1/Subsystem ==
  note: PI CONTROLLER
  note: Wm(N)
  note: Wm(N-1)
  note: Wm(N)
  note: Te(N)
  note: Te(N)*
  note: Te(N-1)*
  We : Inport
  Gain : Gain  Gain=Ki
  Gain1 : Gain  Gain=Kp
  Saturation : Saturate  UpperLimit=Lim  LowerLimit=-Lim
  Sum : Sum  Inputs=|+-
  Sum1 : Sum  Inputs=|++
  Sum2 : Sum  Inputs=|++
  Unit Delay : UnitDelay  SampleTime=Ts  HasFrameUpgradeWarning=on
  Unit Delay1 : UnitDelay  SampleTime=Ts  HasFrameUpgradeWarning=on
  Te* : Outport
  wires:
  Sum1/1 -> Sum2/1
  Sum2/1 -> Saturation/1
  Saturation/1 -> Unit Delay/1, Te*/1
  Sum/1 -> Gain1/1
  Gain1/1 -> Sum1/1
  Unit Delay1/1 -> Sum/2
  We/1 -> Sum/1, Unit Delay1/1, Gain/1
  Gain/1 -> Sum1/2
  Unit Delay/1 -> Sum2/2

== system PV_fed_VCIMD_updated/Conditioning Circuit/PWM modulator/Comparator ==
  In1 : Inport
  In2 : Inport  Port=2
  Constant : Constant
  Constant1 : Constant  Value=0
  Sum : Sum  Inputs=|+-
  Switch : Switch
  Out1 : Outport
  wires:
  Constant1/1 -> Switch/3
  Constant/1 -> Switch/1
  Sum/1 -> Switch/2
  In1/1 -> Sum/1
  Switch/1 -> Out1/1
  In2/1 -> Sum/2

== system PV_fed_VCIMD_updated/Conditioning Circuit/PWM modulator/Sawtooth ==
  Add : Sum  Inputs=+-
  Constant : Constant  Value=.5
  Signal Generator : SignalGenerator  WaveForm=sawtooth  Amplitude=.5  Frequency=10000
  Out1 : Outport
  wires:
  Constant/1 -> Add/1
  Signal Generator/1 -> Add/2
  Add/1 -> Out1/1

== matlab function PV_fed_VCIMD_updated/Conditioning Circuit/Variable DC to Fixed DC ==
  settings: updateMethod=DISCRETE
  data: D output; Vdc input; t1 input
function D = Var2Fix(Vdc, t1)

Vdc_ref = 560.45;

persistent Dold

if isempty(Dold)
    Dold = 0;
end

Dmax = 0.75; Dmin = 0.35;

deltaD = 1e-3;

if t1 < 0.5
    D = 0;
elseif t1 < 1.7
    D = 0.55*(t1-0.5);
else
    if Vdc < Vdc_ref
        D = Dold + deltaD;
    elseif Vdc > Vdc_ref
        D = Dold - deltaD;
    else
        D = Dold;
    end
    
    if D >= Dmax || D <= Dmin
        D=Dold;
    end
end

Dold = D;

== matlab function PV_fed_VCIMD_updated/FEILD WEAKENING ==
  data: wm input; imr output
function imr = fcn(wm)
%#codegen
if wm<2*pi*50
   imr=21.6;
else
    imr=2*pi*50*21.6/wm;
end

== matlab function PV_fed_VCIMD_updated/Conditioning Circuit/MPPT ==
  data: V input; Vmp output; I input
function Vmp = MPPT(V, I)

persistent Vmp_old Pold Vold

if isempty(Vold)
    Vmp_old = 0;
    Pold = 0;
    Vold = 0;
end

deltaV = 0.1;

P = V * I;
dV = V - Vold;
dP = P - Pold;

if abs(dP) <= 100
    if (dP/dV) > 0
        Vmp = Vmp_old + deltaV;
    else
        Vmp = Vmp_old - deltaV;
    end
else
    Vmp = Vmp_old;
end

if Vmp >= 750 || Vmp <= 0
    Vmp = Vmp_old;
end

Vmp_old = Vmp;
Vold = V;
Pold = P;
